simulink model "hw_7"  (R2016b)
settings: Solver=VariableStepAuto  StartTime=0.0  StopTime=10  RelTol=1e-3
libraries: simulink x1
settings Model: Creator=grahamgrable  LastModifiedBy=grahamgrable

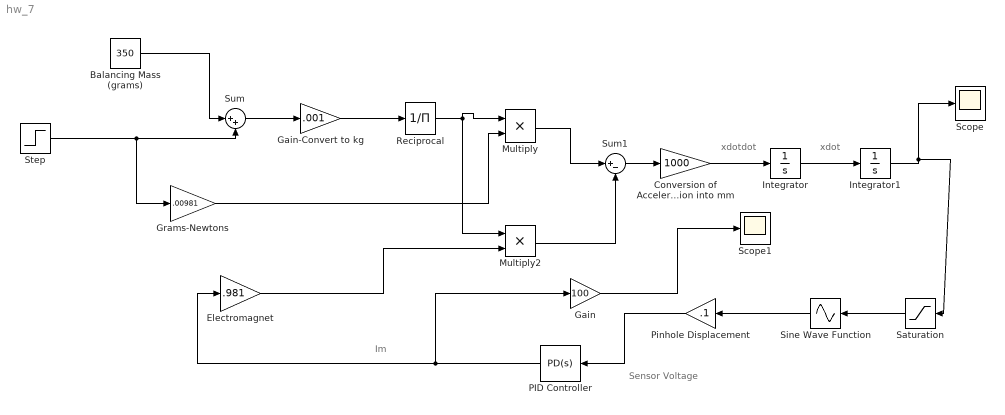
== system hw_7 ==
  note: Im
  note: Sensor Voltage
  note: xdot
  note: xdotdot
  Balancing Mass (grams) : Constant  Value=350
  Conversion of Acceleration into mm : Gain  Gain=1000
  Electromagnet : Gain  Gain=.981
  Gain : Gain  Gain=100
  Gain-Convert to kg : Gain  Gain=.001
  Grams-Newtons : Gain  Gain=.00981
  Integrator : Integrator
  Integrator1 : Integrator
  "Multiply " : Product  Inputs=**
  "Multiply2 " : Product  Inputs=**
  PID Controller : simulink/Continuous/PID Controller  Controller=PD  TimeDomain=Continuous-time  SampleTime=-1  IntegratorMethod=Forward Euler  FilterMethod=Forward Euler  Form=Parallel  UseFilter=on  ControllerParametersSource=internal  P=100  I=1  D=5  N=114.28279760416  InitialConditionSource=internal  InitialConditionForIntegrator=0  InitialConditionForFilter=0  ExternalReset=none  LimitOutput=off  UpperSaturationLimit=inf  LowerSaturationLimit=-inf  LinearizeAsGain=on  AntiWindupMode=none  Kb=1  TrackingMode=off  Kt=1  PParamMin=[]  PParamMax=[]  IParamMin=[]  IParamMax=[]  DParamMin=[]  DParamMax=[]  NParamMin=[]  NParamMax=[]  KbParamMin=[]  KbParamMax=[]  KtParamMin=[]  KtParamMax=[]  POutMin=[]  POutMax=[]  IOutMin=[]  IOutMax=[]  DOutMin=[]  DOutMax=[]  NOutMin=[]  NOutMax=[]  KbOutMin=[]  KbOutMax=[]  KtOutMin=[]  KtOutMax=[]  IntegratorOutMin=[]  IntegratorOutMax=[]  FilterOutMin=[]  FilterOutMax=[]  SumOutMin=[]  SumOutMax=[]  SumI1OutMin=[]  SumI1OutMax=[]  SumI2OutMin=[]  SumI2OutMax=[]  SumI3OutMin=[]  SumI3OutMax=[]  SumDOutMin=[]  SumDOutMax=[]  SaturationOutMin=[]  SaturationOutMax=[]  IntegratorContinuousStateAttributes=''  IntegratorStateMustResolveToSignalObject=off  IntegratorRTWStateStorageClass=Auto  FilterContinuousStateAttributes=''  FilterStateMustResolveToSignalObject=off  FilterRTWStateStorageClass=Auto  DifferentiatorICPrevScaledInput=0  DifferentiatorOutMin=[]  DifferentiatorOutMax=[]
  Pinhole Displacement : Gain  Gain=.1
  Reciprocal : Product  Inputs=/  SaturateOnIntegerOverflow=on  RndMeth=Zero
  Saturation : Saturate  UpperLimit=.785  LowerLimit=-.785
  Scope : Scope
  Scope1 : Scope
  Sine Wave Function : Sin  TimeSource=Use external signal  SampleTime=0
  Step : Step  Time=.1  After=200  SampleTime=.1
  Sum : Sum  Inputs=|++
  Sum1 : Sum  Inputs=|+-
  wires:
  Step/1 -> Grams-Newtons/1, Sum/2
  Balancing Mass (grams)/1 -> Sum/1
  Sum/1 -> Gain-Convert to kg/1
  "Multiply "/1 -> Sum1/1
  Sum1/1 -> Conversion of Acceleration into mm/1
  "Multiply2 "/1 -> Sum1/2
  Electromagnet/1 -> "Multiply2 "/2
  Grams-Newtons/1 -> "Multiply "/2
  Conversion of Acceleration into mm/1 -> Integrator/1
  Integrator/1 -> Integrator1/1
  Integrator1/1 -> Scope/1, Saturation/1
  Saturation/1 -> Sine Wave Function/1
  PID Controller/1 -> Gain/1, Electromagnet/1
  Pinhole Displacement/1 -> PID Controller/1
  Sine Wave Function/1 -> Pinhole Displacement/1
  Reciprocal/1 -> "Multiply "/1, "Multiply2 "/1
  Gain-Convert to kg/1 -> Reciprocal/1
  Gain/1 -> Scope1/1
